simulink model "relay_feedback_with_positive_loop"  (R2015a)
settings: Solver=ode45  StartTime=0.0  StopTime=tmax  RelTol=1e-3
values from neighbouring files (symbols this model uses):
  b = 1    [testing_relay_plant_positive_feedback.m]    (also in testing_simple_relay_hysteresis.m = 1.5; testing_simple_relay_plant.m)
  d = 1    [testing_relay_plant_positive_feedback.m]    (also in testing_simple_relay_hysteresis.m = 2; testing_simple_relay_plant.m)
settings Model: Creator=ra428  LastModifiedBy=ra428

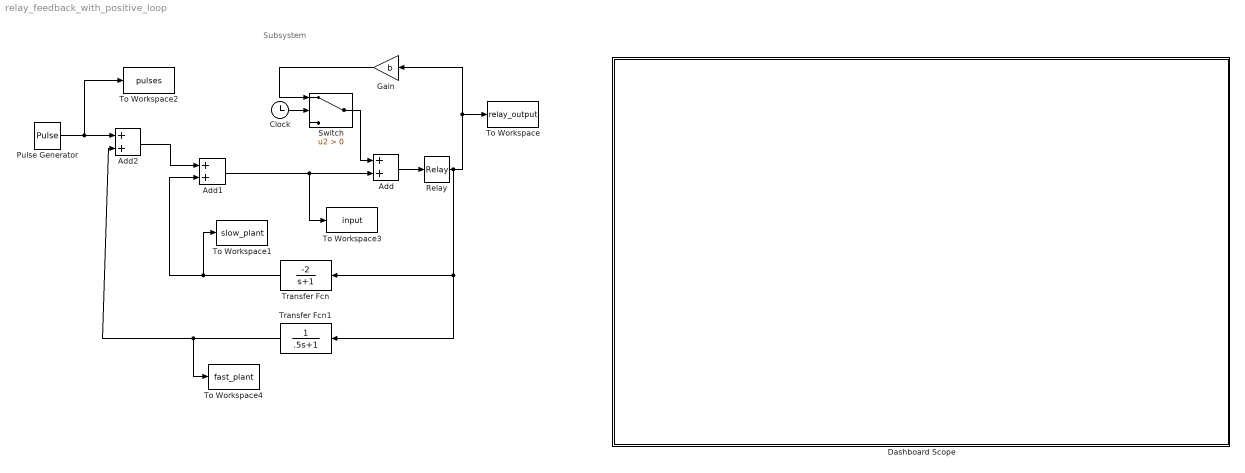
== system relay_feedback_with_positive_loop ==
  note: Subsystem
  Add : Sum
  Add1 : Sum
  Add2 : Sum
  Clock : Clock
  Dashboard Scope : Subsystem  DialogController=hmiCreateDDGDialog  IsWebBlock=on  mask(MathWorksWebBlock){webBlockId=4b2ea97f-dbcc-4152-9b11-5e345150a749, webBlockType=sdiscope, ShowInitialText=on, HMISrcModelName=relay_feedback_with_positive_loop}
      mask prompts: webBlockId "WebBlock Id"; webBlockType "WebBlock Type"; HMISrcModelName "Source Model"
      mask Help: helpview([docroot '/mapfiles/simulink.map'], 'hmi_scope')
      mask Display:
      | if strcmp(get_param(bdroot(gcb),'BlockDiagramType'), 'library')
      |     image([(matlabroot) '/toolbox/simulink/hmi/icons/DashboardScope.png']);
      | end
  Gain : Gain  Gain=b
  Pulse Generator : DiscretePulseGenerator  PulseType=Time based  Period=400  PulseWidth=50  PhaseDelay=200
  Relay : Relay  OnSwitchValue=0  OffSwitchValue=0  OnOutputValue=d  OffOutputValue=-d
  Switch : Switch  Criteria=u2 > Threshold
  To Workspace : ToWorkspace  VariableName=relay_output  SaveFormat=Timeseries  SampleTime=-1
  To Workspace1 : ToWorkspace  VariableName=slow_plant  SaveFormat=Timeseries  SampleTime=-1
  To Workspace2 : ToWorkspace  VariableName=pulses  SaveFormat=Timeseries  SampleTime=-1
  To Workspace3 : ToWorkspace  VariableName=input  SaveFormat=Timeseries  SampleTime=-1
  To Workspace4 : ToWorkspace  VariableName=fast_plant  SaveFormat=Timeseries  SampleTime=-1
  Transfer Fcn : TransferFcn  Numerator=[-2]  Denominator=[1 1]
  Transfer Fcn1 : TransferFcn  Denominator=[.5 1]
  wires:
  Transfer Fcn/1 -> Add1/2, To Workspace1/1
  Pulse Generator/1 -> Add2/1, To Workspace2/1
  Transfer Fcn1/1 -> To Workspace4/1, Add2/2
  Add2/1 -> Add1/1
  Relay/1 -> To Workspace/1, Gain/1, Transfer Fcn1/1, Transfer Fcn/1
  Add/1 -> Relay/1
  Switch/1 -> Add/1
  Add1/1 -> To Workspace3/1, Add/2
  Gain/1 -> Switch/1
  ? -> Switch/3
  Clock/1 -> Switch/2

== system relay_feedback_with_positive_loop/Dashboard Scope ==
